simulink model "Quaternions_Method"  (R2021b)
settings: Solver=ode113  StartTime=0.0  StopTime=Time  RelTol=1e-13  AbsTol=1e-8
undefined symbols (not defined in the file): a, A_MB, A_SP, c, e, I, ii, Iinv, Ix, Iy, Iz, muP, om_x, om_y, om_z, omega_0, RS_MB, Rs_SP, theta00
libraries: vrlib x3, matrix_library x3, simulink_extras x1, robotcorelib x1
settings Model: Creator=dario  LastModifiedBy=adity
settings SolverCC: InitialStep=1e-3  AlgebraicLoopSolver=TrustRegion

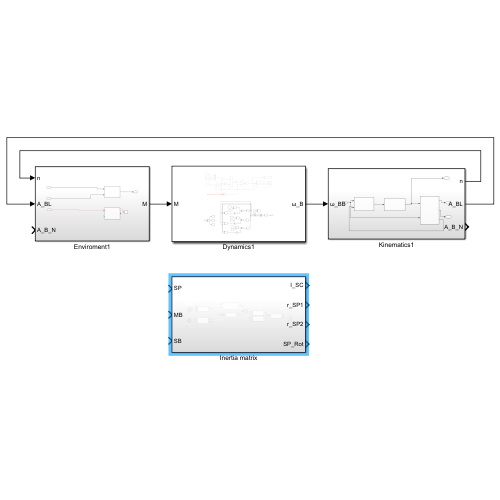
[thumbnail: Simulink's stored preview of the top-level diagram]
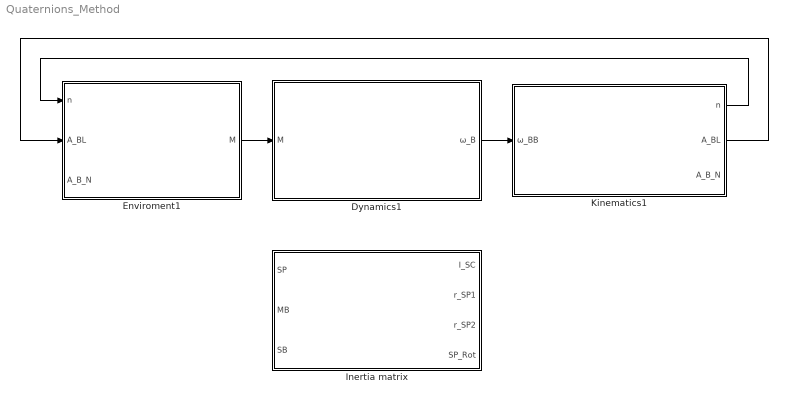
== system Quaternions_Method ==
  Dynamics1 : Subsystem
  Enviroment1 : Subsystem
  Inertia matrix : Subsystem
  Kinematics1 : Subsystem
  wires:
  Kinematics1/1(n) -> Enviroment1/1(n)
  Kinematics1/2(A_BL) -> Enviroment1/2(A_BL)
  Dynamics1/1(ω_B) -> Kinematics1/1(ω_BB)
  Enviroment1/1(M) -> Dynamics1/1(M)

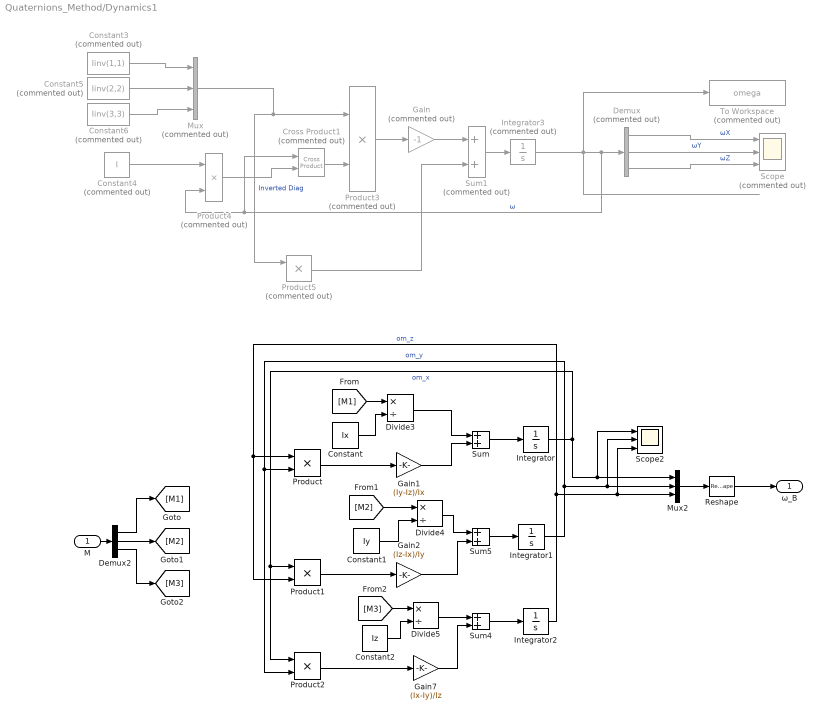
== system Quaternions_Method/Dynamics1 ==
  M : Inport
  Constant : Constant  Value=Ix
  Constant1 : Constant  Value=Iy
  Constant2 : Constant  Value=Iz
  Constant3 : Constant  Commented=on  Value=Iinv(1,1)
  Constant4 : Constant  Commented=on  Value=I
  Constant5 : Constant  Commented=on  Value=Iinv(2,2)
  Constant6 : Constant  Commented=on  Value=Iinv(3,3)
  Cross Product1 : vrlib/Utilities/Cross Product  Commented=on
  Demux : Demux  Commented=on  Outputs=3
  Demux2 : Demux  Outputs=3
  Divide3 : Product  Inputs=*/
  Divide4 : Product  Inputs=*/
  Divide5 : Product  Inputs=*/
  Gain : Gain  Commented=on  Gain=-1
  Gain1 : Gain  Gain=(Iy-Iz)/Ix
  Gain2 : Gain  Gain=(Iz-Ix)/Iy
  Gain7 : Gain  Gain=(Ix-Iy)/Iz
  Integrator : Integrator  InitialCondition=om_x
  Integrator1 : Integrator  InitialCondition=om_y
  Integrator2 : Integrator  InitialCondition=om_z
  Integrator3 : Integrator  Commented=on  InitialCondition=omega_0
  Mux : Mux  Commented=on  Inputs=3
  Mux2 : Mux  Inputs=3
  Product : Product
  Product1 : Product
  Product2 : Product
  Product3 : Product  Commented=on
  Product4 : Product  Commented=on
  Product5 : Product  Commented=on
  Reshape : Reshape  OutputDimensionality=Column vector (2-D)
  Scope : Scope  Commented=on  NumInputPorts=3
  Scope2 : Scope  NumInputPorts=3
  Sum : Sum  Inputs=|+|+|
  Sum1 : Sum  Commented=on
  Sum4 : Sum  Inputs=|+|+|
  Sum5 : Sum  Inputs=|+|+|
  To Workspace : ToWorkspace  Commented=on  VariableName=omega  SaveFormat=Timeseries  SampleTime=-1
  ω_B : Outport
  wires:
  Demux2/2 -> [M2]
  Demux2/3 -> [M3]
  Demux2/1 -> [M1]
  M/1 -> Demux2/1
  Integrator/1 -> Product2/1, Product1/1, Scope2/1, Mux2/1  "om_x"
  Integrator1/1 -> Scope2/2, Mux2/2, Product2/2, Product/2  "om_y"
  Integrator2/1 -> Mux2/3, Scope2/3, Product1/2, Product/1  "om_z"
  [M1] -> Divide3/1
  Constant/1 -> Divide3/2
  Product/1 -> Gain1/1
  Gain1/1 -> Sum/2
  Divide3/1 -> Sum/1
  Sum/1 -> Integrator/1
  [M2] -> Divide4/1
  Constant1/1 -> Divide4/2
  Divide4/1 -> Sum5/1
  Product1/1 -> Gain2/1
  Gain2/1 -> Sum5/2
  Sum5/1 -> Integrator1/1
  [M3] -> Divide5/1
  Constant2/1 -> Divide5/2
  Divide5/1 -> Sum4/1
  Sum4/1 -> Integrator2/1
  Product2/1 -> Gain7/1
  Gain7/1 -> Sum4/2
  Integrator3/1 -> To Workspace/1, Demux/1, Product4/2, Cross Product1/1  "ω"
  Sum1/1 -> Integrator3/1
  Mux/1 -> Product5/1, Product3/1  "Inverted Diag"
  Constant6/1 -> Mux/3
  Gain/1 -> Sum1/1
  Cross Product1/1 -> Product3/2
  Product3/1 -> Gain/1
  ? -> Product5/2
  Product5/1 -> Sum1/2
  Demux/2 -> Scope/2  "ωY"
  Constant3/1 -> Mux/1
  Constant5/1 -> Mux/2
  Product4/1 -> Cross Product1/2
  Constant4/1 -> Product4/1
  Demux/1 -> Scope/1  "ωX"
  Demux/3 -> Scope/3  "ωZ"
  Mux2/1 -> Reshape/1
  Reshape/1 -> ω_B/1

== system Quaternions_Method/Enviroment1 ==
  n : Inport
  A_BL : Inport  Port=2
  A_B_N : Inport  Port=3
  Gravity_Gradient : Subsystem
  Solar Radiation Perturbation : Subsystem
  Terminator : Terminator
  M : Outport
  wires:
  A_BL/1 -> Gravity_Gradient/1(A_BL)
  Gravity_Gradient/1(M_GG) -> M/1
  n/1 -> Gravity_Gradient/2(n)
  ? -> Terminator/1
  A_B_N/1 -> ?

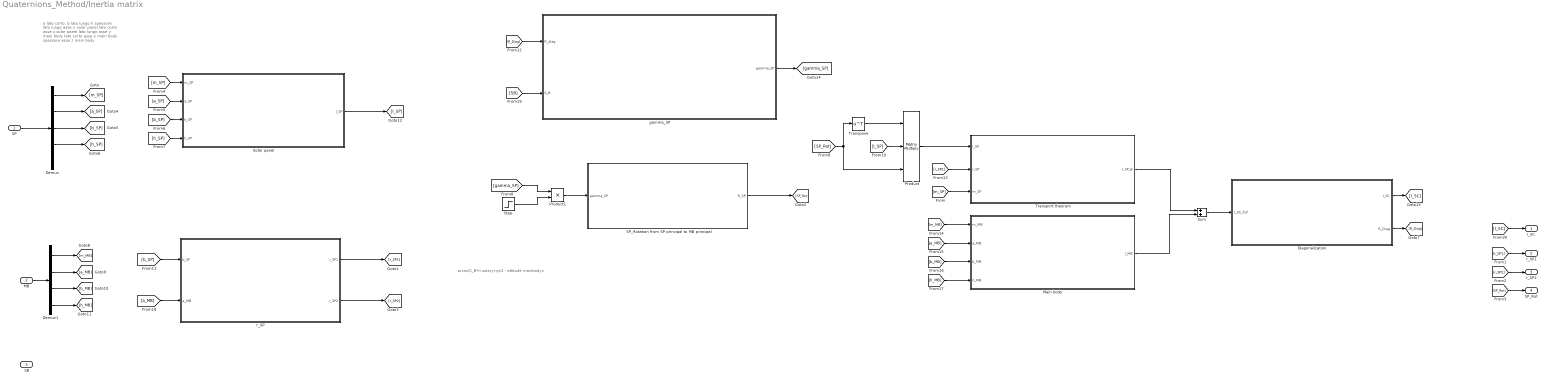
== system Quaternions_Method/Inertia matrix ==
  note: arcos(S_B*n solary)-pi/2 - attitude mainbodyx
  note: a lato corto, b lato lungo h spessore
      | lato lungo asse x solar panel
      | lato corto asse z solar panel
      | lato lungo asse y main body
      | lato corto asse x main body
      | spessore asse z main body
  SP : Inport
  MB : Inport  Port=2
  SB : Inport  Port=3
  Demux : Demux  Outputs=5
  Demux1 : Demux
  Diagonalization : Subsystem
  Main body : Subsystem
  Product : Product  Inputs=3  Multiplication=Matrix(*)
  Product1 : Product
  SP_Rotation from SP principal to MB principal : Subsystem
  Solar panel : Subsystem
  Step : Step  Time=1e-3  SampleTime=0
  Sum : Sum
  Transport theorem : Subsystem
  Transpose : Math  Operator=transpose  SaturateOnIntegerOverflow=on
  gamma_SP : Subsystem
  r_SP : Subsystem
  I_SC : Outport
  r_SP1 : Outport  Port=2
  r_SP2 : Outport  Port=3
  SP_Rot : Outport  Port=4
  wires:
  MB/1 -> Demux1/1
  Demux/1 -> [m_SP]
  Product/1 -> Transport theorem/1(I_SP)
  SP_Rotation from SP principal to MB principal/1(R_SP) -> [SP_Rot]
  Transpose/1 -> Product/1
  Transport theorem/1(I_SP_B) -> Sum/1
  [r_SP1] -> Transport theorem/2(r_SP)
  Sum/1 -> Diagonalization/1(I_SC_full)
  Main body/1(I_MB) -> Sum/2
  [m_SP] -> Transport theorem/3(m_SP)
  r_SP/1(r_SP1) -> [r_SP1]
  [r_SP1] -> r_SP1/1
  [r_SP2] -> r_SP2/1
  [SP_Rot] -> SP_Rot/1
  r_SP/2(r_SP2) -> [r_SP2]
  Demux/2 -> [a_SP]
  Demux/3 -> [b_SP]
  Demux/4 -> [h_SP]
  [a_SP] -> Solar panel/2(a_SP)
  [b_SP] -> Solar panel/3(b_SP)
  [m_SP] -> Solar panel/1(m_SP)
  [h_SP] -> Solar panel/4(h_SP)
  [SP_Rot] -> Transpose/1, Product/3
  [b_SP] -> r_SP/1(b_SP)
  Demux1/4 -> [h_MB]
  Demux1/3 -> [b_MB]
  Demux1/2 -> [a_MB]
  Demux1/1 -> [m_MB]
  [m_MB] -> Main body/1(m_MB)
  [a_MB] -> Main body/2(a_MB)
  [b_MB] -> Main body/3(b_MB)
  [h_MB] -> Main body/4(h_MB)
  [a_MB] -> r_SP/2(a_MB)
  Solar panel/1(I_SP) -> [I_SP]
  [I_SP] -> Product/2
  Product1/1 -> SP_Rotation from SP principal to MB principal/1(gamma_SP)
  [gamma_SP] -> Product1/1
  Step/1 -> Product1/2
  SP/1 -> Demux/1
  Diagonalization/2(R_Diag) -> [R_Diag]
  [R_Diag] -> gamma_SP/1(R_diag)
  [SB] -> gamma_SP/2(S_B)
  Diagonalization/1(I_SC) -> [I_SC]
  [I_SC] -> I_SC/1
  gamma_SP/1(gamma_SP) -> [gamma_SP]

== system Quaternions_Method/Kinematics1 ==
  ω_BB : Inport
  Creazione Matrice A_BN : Subsystem
  Creazione quaternione : Subsystem
  Relative_Attitude : Subsystem
  n : Outport
  A_BL : Outport  Port=2
  A_B_N : Outport  Port=3
  wires:
  Creazione Matrice A_BN/1(A_BN) -> A_B_N/1, Relative_Attitude/1(A_BN)
  ω_BB/1 -> Relative_Attitude/2(ω_BB), Creazione quaternione/1(ω_BB)
  Creazione quaternione/1(q_normalizzato) -> Creazione Matrice A_BN/1(q_normalizzato)
  Relative_Attitude/1(A_BL) -> A_BL/1
  Relative_Attitude/2(n) -> n/1
  Relative_Attitude/3(A_L/N) -> Creazione quaternione/2(A_LN)

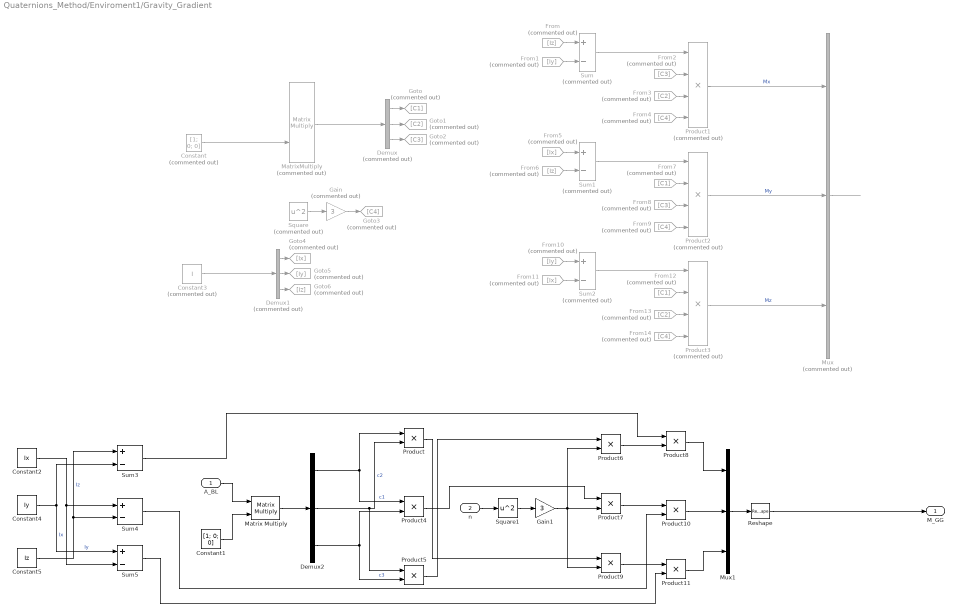
== system Quaternions_Method/Enviroment1/Gravity_Gradient ==
  A_BL : Inport
  n : Inport  Port=2
  Constant : Constant  Commented=on  Value=[1; 0; 0]
  Constant1 : Constant  Value=[1; 0; 0]
  Constant2 : Constant  Value=Ix
  Constant3 : Constant  Commented=on  Value=I
  Constant4 : Constant  Value=Iy
  Constant5 : Constant  Value=Iz
  Demux : Demux  Commented=on  Outputs=3
  Demux1 : Demux  Commented=on  Outputs=3
  Demux2 : Demux  Outputs=3
  From : From  Commented=on  GotoTag=Iz
  From1 : From  Commented=on  GotoTag=Iy
  From10 : From  Commented=on  GotoTag=Iy
  From11 : From  Commented=on  GotoTag=Ix
  From12 : From  Commented=on  GotoTag=C1
  From13 : From  Commented=on  GotoTag=C2
  From14 : From  Commented=on  GotoTag=C4
  From2 : From  Commented=on  GotoTag=C3
  From3 : From  Commented=on  GotoTag=C2
  From4 : From  Commented=on  GotoTag=C4
  From5 : From  Commented=on  GotoTag=Ix
  From6 : From  Commented=on  GotoTag=Iz
  From7 : From  Commented=on  GotoTag=C1
  From8 : From  Commented=on  GotoTag=C3
  From9 : From  Commented=on  GotoTag=C4
  Gain : Gain  Commented=on  Gain=3
  Gain1 : Gain  Gain=3
  Goto : Goto  Commented=on  GotoTag=C1
  Goto1 : Goto  Commented=on  GotoTag=C2
  Goto2 : Goto  Commented=on  GotoTag=C3
  Goto3 : Goto  Commented=on  GotoTag=C4
  Goto4 : Goto  Commented=on  GotoTag=Ix
  Goto5 : Goto  Commented=on  GotoTag=Iy
  Goto6 : Goto  Commented=on  GotoTag=Iz
  Matrix Multiply : Product  Multiplication=Matrix(*)
  MatrixMultiply : Product  Commented=on  Multiplication=Matrix(*)
  Mux : Mux  Commented=on  Inputs=3
  Mux1 : Mux  Inputs=3
  Product{,4..11} (9 alike) : Product
  Product1 : Product  Commented=on  Inputs=4
  Product2 : Product  Commented=on  Inputs=4
  Product3 : Product  Commented=on  Inputs=4
  Reshape : Reshape  OutputDimensionality=Column vector (2-D)
  Square : Math  Commented=on  Operator=square  SaturateOnIntegerOverflow=on
  Square1 : Math  Operator=square  SaturateOnIntegerOverflow=on
  Sum : Sum  Commented=on  Inputs=+-
  Sum1 : Sum  Commented=on  Inputs=+-
  Sum2 : Sum  Commented=on  Inputs=+-
  Sum3 : Sum  Inputs=|+|-|
  Sum4 : Sum  Inputs=|+|-|
  Sum5 : Sum  Inputs=|+|-|
  M_GG : Outport
  wires:
  Constant/1 -> MatrixMultiply/2
  MatrixMultiply/1 -> Demux/1
  Constant3/1 -> Demux1/1
  Product1/1 -> Mux/1  "Mx"
  Product2/1 -> Mux/2  "My"
  Demux/1 -> Goto/1
  Demux/2 -> Goto1/1
  Demux/3 -> Goto2/1
  Demux1/1 -> Goto4/1
  Demux1/2 -> Goto5/1
  Demux1/3 -> Goto6/1
  From/1 -> Sum/1
  From1/1 -> Sum/2
  Sum/1 -> Product1/1
  From2/1 -> Product1/2
  From3/1 -> Product1/3
  From4/1 -> Product1/4
  From5/1 -> Sum1/1
  From6/1 -> Sum1/2
  Sum1/1 -> Product2/1
  From7/1 -> Product2/2
  From8/1 -> Product2/3
  From9/1 -> Product2/4
  From10/1 -> Sum2/1
  From14/1 -> Product3/4
  From12/1 -> Product3/2
  From13/1 -> Product3/3
  Sum2/1 -> Product3/1
  From11/1 -> Sum2/2
  Product3/1 -> Mux/3  "Mz"
  Square/1 -> Gain/1
  Gain/1 -> Goto3/1
  A_BL/1 -> Matrix Multiply/1
  Constant1/1 -> Matrix Multiply/2
  Matrix Multiply/1 -> Demux2/1
  Demux2/1 -> Product4/1, Product/1  "c1"
  Demux2/3 -> Product5/2, Product4/2  "c3"
  Demux2/2 -> Product5/1, Product/2  "c2"
  Constant5/1 -> Sum4/2, Sum3/1  "Iz"
  Constant4/1 -> Sum3/2, Sum5/1  "Iy"
  Constant2/1 -> Sum5/2, Sum4/1  "Ix"
  n/1 -> Square1/1
  Square1/1 -> Gain1/1
  Product5/1 -> Product6/1
  Gain1/1 -> Product9/2, Product7/2, Product6/2
  Product4/1 -> Product7/1
  Product/1 -> Product9/1
  Sum3/1 -> Product8/1
  Product6/1 -> Product8/2
  Product7/1 -> Product10/1
  Sum4/1 -> Product10/2
  Sum5/1 -> Product11/2
  Product9/1 -> Product11/1
  Product10/1 -> Mux1/2
  Product8/1 -> Mux1/1
  Product11/1 -> Mux1/3
  ? -> MatrixMultiply/1
  ? -> Square/1
  Mux/1 -> ?
  Mux1/1 -> Reshape/1
  Reshape/1 -> M_GG/1

== system Quaternions_Method/Enviroment1/Solar Radiation Perturbation ==
  n_SP : Inport
  A_B_N : Inport  Port=2
  Constant : Constant  Value=A_SP
  Constant1 : Constant  Value=Rs_SP
  Constant2 : Constant  Value=RS_MB
  Constant3 : Constant  Value=A_MB
  Constant6 : Constant  Value=1358
  Constant7 : Constant  Value=c
  Force : Subsystem
  From Workspace1 : FromWorkspace  VariableName=Rd
  N_MB : Constant  Value=[1 0 0;0 1 0;0 0 1]
  Normalize Vector : vrlib/Utilities/Normalize Vector  maxzero=0
  Product : Product
  Reciprocal : Product  Inputs=1
  Sum forces : Subsystem
  Sun position body : Subsystem
  Output : Outport
  wires:
  From Workspace1/1 -> Force/9(R_D)
  Constant/1 -> Force/7(A_SP)
  n_SP/1 -> Force/6(n_SP)
  Constant7/1 -> Reciprocal/1
  Constant6/1 -> Product/1
  Constant3/1 -> Force/3(A_MB)
  Constant2/1 -> Force/2(RS_MB)
  N_MB/1 -> Force/5(N_MB)
  Constant1/1 -> Force/8(Rs_SP)
  Normalize Vector/1 -> Force/4(SB)
  Reciprocal/1 -> Product/2
  Product/1 -> Force/1(P)
  A_B_N/1 -> Sun position body/1(A_B_N)
  Sun position body/1(S_B) -> Normalize Vector/1

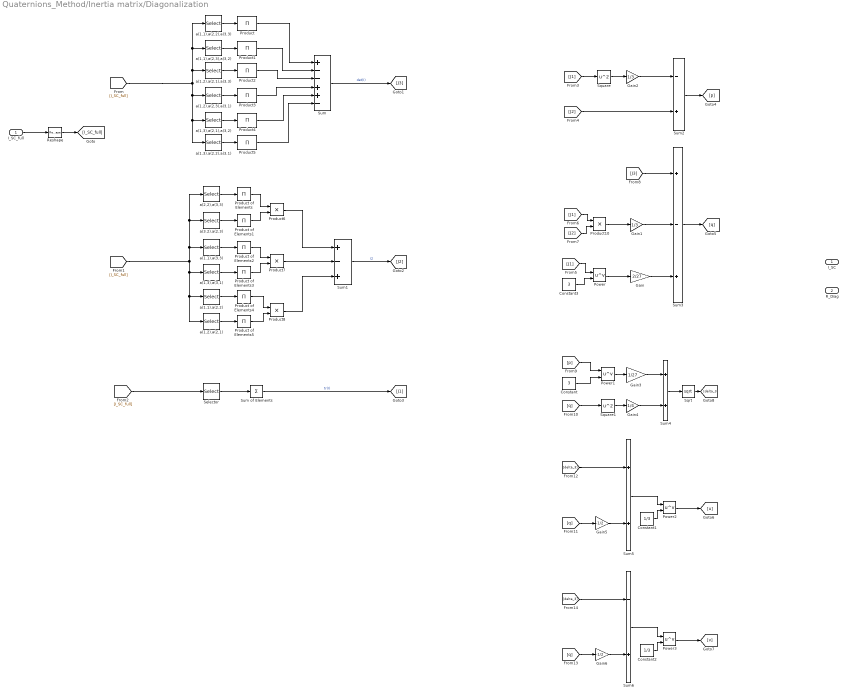
== system Quaternions_Method/Inertia matrix/Diagonalization ==
  I_SC_full : Inport
  Constant : Constant  Value=3
  Constant1 : Constant  Value=1/3
  Constant2 : Constant  Value=1/3
  Constant3 : Constant  Value=3
  Gain : Gain  Gain=2/27
  Gain1 : Gain  Gain=1/3
  Gain2 : Gain  Gain=1/3
  Gain3 : Gain  Gain=1/27
  Gain4 : Gain  Gain=1/4
  Gain5 : Gain  Gain=-1/2
  Gain6 : Gain  Gain=-1/2
  Power{,1..3} (4 alike) : Math  Operator=pow  SaturateOnIntegerOverflow=on
  Product{,1..5} (6 alike) : Product  Inputs=1  SaturateOnIntegerOverflow=on  OutDataTypeStr=Inherit: Same as first input
  Product of Elements{,1..5} (6 alike) : Product  Inputs=*
  Product{6..8,10} (4 alike) : Product
  Reshape : Reshape  OutputDimensionality=Column vector (2-D)
  Selector : Selector  InputPortWidth=9  IndexOptions=Index vector (dialog)  Indices=[1 5 9]  OutputSizes=1
  Sqrt : Sqrt  SaturateOnIntegerOverflow=on
  Square : Math  Operator=square  SaturateOnIntegerOverflow=on
  Square1 : Math  Operator=square  SaturateOnIntegerOverflow=on
  Sum : Sum  Inputs=+--++-  SaturateOnIntegerOverflow=on
  Sum of Elements : Sum  Inputs=+
  Sum1 : Sum  Inputs=+-+
  Sum2 : Sum  Inputs=-+
  Sum3 : Sum  Inputs=+-+
  Sum4 : Sum
  Sum5 : Sum
  Sum6 : Sum  Inputs=-+
  a(1,1),a(2,2) : Selector  InputPortWidth=9  IndexOptions=Index vector (dialog)  Indices=[1 3]  OutputSizes=1
  a(1,1),a(2,2),a(3,3) : Selector  InputPortWidth=9  IndexOptions=Index vector (dialog)  Indices=[1 5 9]  OutputSizes=1
  a(1,1),a(2,3),a(3,2) : Selector  InputPortWidth=9  IndexOptions=Index vector (dialog)  Indices=[1 6 8]  OutputSizes=1
  a(1,2),a(2,1) : Selector  InputPortWidth=9  IndexOptions=Index vector (dialog)  Indices=[1 3]  OutputSizes=1
  a(1,2),a(2,1),a(3,3) : Selector  InputPortWidth=9  IndexOptions=Index vector (dialog)  Indices=[2 4 9]  OutputSizes=1
  a(1,2),a(2,3),a(3,1) : Selector  InputPortWidth=9  IndexOptions=Index vector (dialog)  Indices=[3 4 8]  OutputSizes=1
  a(1,3),a(2,1),a(3,2) : Selector  InputPortWidth=9  IndexOptions=Index vector (dialog)  Indices=[2 6 7]  OutputSizes=1
  a(1,3),a(2,2),a(3,1) : Selector  InputPortWidth=9  IndexOptions=Index vector (dialog)  Indices=[3 5 7]  OutputSizes=1
  a(1,3),a(3,1) : Selector  InputPortWidth=9  IndexOptions=Index vector (dialog)  Indices=[1 3]  OutputSizes=1
  a(1.1),a(3,3) : Selector  InputPortWidth=9  IndexOptions=Index vector (dialog)  Indices=[1 3]  OutputSizes=1
  a(2,2),a(3,3) : Selector  InputPortWidth=9  IndexOptions=Index vector (dialog)  Indices=[5 9]  OutputSizes=1
  a(3.2),a(2,3) : Selector  InputPortWidth=9  IndexOptions=Index vector (dialog)  Indices=[6 8]  OutputSizes=1
  I_SC : Outport
  R_Diag : Outport  Port=2
  wires:
  [I_SC_full] -> a(1,3),a(2,2),a(3,1)/1, a(1,3),a(2,1),a(3,2)/1, a(1,2),a(2,3),a(3,1)/1, a(1,1),a(2,2),a(3,3)/1, a(1,1),a(2,3),a(3,2)/1, a(1,2),a(2,1),a(3,3)/1
  Product2/1 -> Sum/3
  Product3/1 -> Sum/4
  a(1,2),a(2,1),a(3,3)/1 -> Product2/1
  a(1,1),a(2,3),a(3,2)/1 -> Product1/1
  Product/1 -> Sum/1
  a(1,3),a(2,2),a(3,1)/1 -> Product5/1
  a(1,1),a(2,2),a(3,3)/1 -> Product/1
  a(1,3),a(2,1),a(3,2)/1 -> Product4/1
  Product4/1 -> Sum/5
  Product1/1 -> Sum/2
  Product5/1 -> Sum/6
  a(1,2),a(2,3),a(3,1)/1 -> Product3/1
  I_SC_full/1 -> Reshape/1
  Reshape/1 -> [I_SC_full]
  Sum/1 -> [J3]  "det(I)"
  Product6/1 -> Sum1/1
  Product7/1 -> Sum1/2
  Product8/1 -> Sum1/3
  Sum1/1 -> [J2]  "I2"
  [I_SC_full] -> a(1,3),a(3,1)/1, a(1,1),a(2,2)/1, a(1,2),a(2,1)/1, a(1.1),a(3,3)/1, a(3.2),a(2,3)/1, a(2,2),a(3,3)/1
  [I_SC_full] -> Selector/1
  Selector/1 -> Sum of Elements/1
  a(2,2),a(3,3)/1 -> Product of Elements/1
  a(3.2),a(2,3)/1 -> Product of Elements1/1
  a(1.1),a(3,3)/1 -> Product of Elements2/1
  a(1,3),a(3,1)/1 -> Product of Elements3/1
  a(1,1),a(2,2)/1 -> Product of Elements4/1
  a(1,2),a(2,1)/1 -> Product of Elements5/1
  Product of Elements5/1 -> Product8/2
  Product of Elements4/1 -> Product8/1
  Product of Elements3/1 -> Product7/2
  Product of Elements2/1 -> Product7/1
  Product of Elements1/1 -> Product6/2
  Product of Elements/1 -> Product6/1
  Sum of Elements/1 -> [J1]  "tr(I)"
  [J2] -> Sum2/2
  [J1] -> Square/1
  Square/1 -> Gain2/1
  Gain2/1 -> Sum2/1
  Sum2/1 -> [p]
  [J2] -> Product10/2
  [J1] -> Product10/1
  [J3] -> Sum3/1
  Constant3/1 -> Power/2
  [J1] -> Power/1
  Power/1 -> Gain/1
  Product10/1 -> Gain1/1
  Gain1/1 -> Sum3/2
  Gain/1 -> Sum3/3
  Sum3/1 -> [q]
  [q] -> Square1/1
  [p] -> Power1/1
  Constant/1 -> Power1/2
  Square1/1 -> Gain4/1
  Power1/1 -> Gain3/1
  Gain4/1 -> Sum4/2
  Gain3/1 -> Sum4/1
  Sum4/1 -> Sqrt/1
  [q] -> Gain5/1
  Gain5/1 -> Sum5/2
  Sum5/1 -> Power2/1
  Constant1/1 -> Power2/2
  Power2/1 -> [u]
  Sqrt/1 -> [delta_3]
  [delta_3] -> Sum5/1
  [delta_3] -> Sum6/1
  Constant2/1 -> Power3/2
  Sum6/1 -> Power3/1
  [q] -> Gain6/1
  Power3/1 -> [v]
  Gain6/1 -> Sum6/2

== system Quaternions_Method/Inertia matrix/Main body ==
  m_MB : Inport
  a_MB : Inport  Port=2
  b_MB : Inport  Port=3
  h_MB : Inport  Port=4
  Gain : Gain  Gain=1/12
  Gain1 : Gain  Gain=1/12
  Gain2 : Gain  Gain=1/12
  Ground : Ground
  Product : Product
  Product1 : Product
  Product2 : Product
  Reshape : Reshape  OutputDimensionality=Customize  OutputDimensions=[3,3]
  Square : Math  Operator=square  SaturateOnIntegerOverflow=on
  Square1 : Math  Operator=square  SaturateOnIntegerOverflow=on
  Square2 : Math  Operator=square  SaturateOnIntegerOverflow=on
  Sum : Sum
  Sum1 : Sum
  Sum2 : Sum
  Vector Concatenate : Concatenate  NumInputs=9
  I_MB : Outport
  wires:
  Ground/1 -> Vector Concatenate/2, Vector Concatenate/3, Vector Concatenate/7, Vector Concatenate/8, Vector Concatenate/6, Vector Concatenate/4
  Square/1 -> Sum2/1, Sum1/1
  Square1/1 -> Sum2/2, Sum/1
  Square2/1 -> Sum/2, Sum1/2
  Product1/1 -> Gain1/1
  Gain/1 -> Vector Concatenate/1
  Product2/1 -> Gain2/1
  Sum1/1 -> Product1/2
  m_MB/1 -> Product/1, Product2/1, Product1/1
  Sum2/1 -> Product2/2
  a_MB/1 -> Square/1
  Vector Concatenate/1 -> Reshape/1
  Sum/1 -> Product/2
  b_MB/1 -> Square1/1
  Gain1/1 -> Vector Concatenate/5
  Product/1 -> Gain/1
  Gain2/1 -> Vector Concatenate/9
  Reshape/1 -> I_MB/1
  h_MB/1 -> Square2/1

== system Quaternions_Method/Inertia matrix/SP_Rotation from SP principal to MB principal ==
  gamma_SP : Inport
  Constant : Constant
  Gain : Gain  Gain=-1
  Ground : Ground
  Reshape : Reshape  OutputDimensionality=Customize  OutputDimensions=[3,3]
  Sin : Trigonometry  Operator=cos
  Sin1 : Trigonometry
  Vector Concatenate : Concatenate  NumInputs=9
  R_SP : Outport
  wires:
  Vector Concatenate/1 -> Reshape/1
  Reshape/1 -> R_SP/1
  Constant/1 -> Vector Concatenate/1
  Ground/1 -> Vector Concatenate/7, Vector Concatenate/4, Vector Concatenate/3, Vector Concatenate/2
  gamma_SP/1 -> Sin1/1, Sin/1
  Gain/1 -> Vector Concatenate/6
  Sin/1 -> Vector Concatenate/5, Vector Concatenate/9
  Sin1/1 -> Gain/1, Vector Concatenate/8

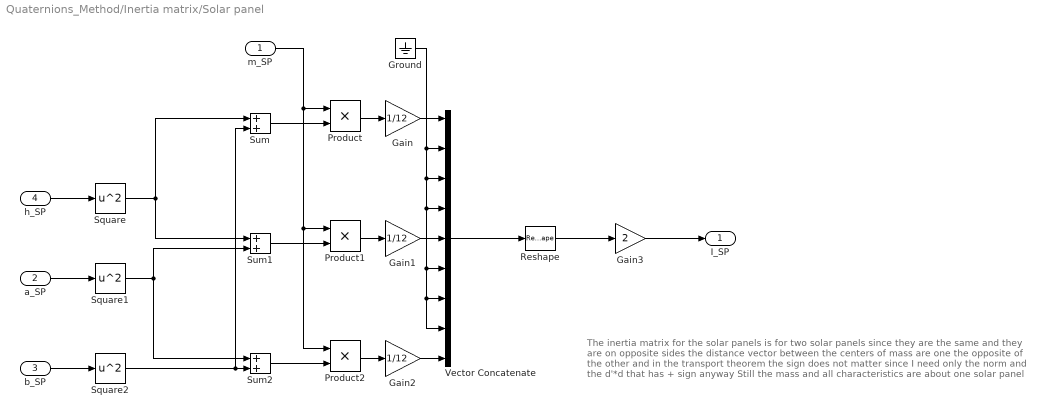
== system Quaternions_Method/Inertia matrix/Solar panel ==
  note: The inertia matrix for the solar panels is for two solar panels since they are the same and they are on opposite sides the distance vector between the centers of mass are one the opposite of the other and in the transport theorem the sign does not matter since I need only the norm and the d'*d that has + sign anyway
      | Still the mass and all characteristics are about one solar panel
  m_SP : Inport
  a_SP : Inport  Port=2
  b_SP : Inport  Port=3
  h_SP : Inport  Port=4
  Gain : Gain  Gain=1/12
  Gain1 : Gain  Gain=1/12
  Gain2 : Gain  Gain=1/12
  Gain3 : Gain  Gain=2
  Ground : Ground
  Product : Product
  Product1 : Product
  Product2 : Product
  Reshape : Reshape  OutputDimensionality=Customize  OutputDimensions=[3,3]
  Square : Math  Operator=square  SaturateOnIntegerOverflow=on
  Square1 : Math  Operator=square  SaturateOnIntegerOverflow=on
  Square2 : Math  Operator=square  SaturateOnIntegerOverflow=on
  Sum : Sum
  Sum1 : Sum
  Sum2 : Sum
  Vector Concatenate : Concatenate  NumInputs=9
  I_SP : Outport
  wires:
  Vector Concatenate/1 -> Reshape/1
  m_SP/1 -> Product/1, Product2/1, Product1/1
  Product/1 -> Gain/1
  Gain/1 -> Vector Concatenate/1
  Product1/1 -> Gain1/1
  Product2/1 -> Gain2/1
  Gain2/1 -> Vector Concatenate/9
  h_SP/1 -> Square/1
  a_SP/1 -> Square1/1
  b_SP/1 -> Square2/1
  Sum/1 -> Product/2
  Sum1/1 -> Product1/2
  Sum2/1 -> Product2/2
  Ground/1 -> Vector Concatenate/2, Vector Concatenate/3, Vector Concatenate/7, Vector Concatenate/8, Vector Concatenate/6, Vector Concatenate/4
  Gain1/1 -> Vector Concatenate/5
  Reshape/1 -> Gain3/1
  Gain3/1 -> I_SP/1
  Square1/1 -> Sum1/2, Sum2/1
  Square2/1 -> Sum/2, Sum2/2
  Square/1 -> Sum/1, Sum1/1

== system Quaternions_Method/Inertia matrix/Transport theorem ==
  I_SP : Inport
  r_SP : Inport  Port=2
  m_SP : Inport  Port=3
  Constant : Constant  Value=eye(3)
  Dot Product : DotProduct  InputSameDT=on  OutDataTypeStr=Inherit: Inherit via internal rule
  Gain : Gain  Gain=2
  Matrix Multiply : Product  Multiplication=Matrix(*)
  Matrix Multiply1 : Product
  Product : Product
  Sum : Sum  Inputs=+-
  Sum1 : Sum
  Transpose : Math  Operator=transpose  SaturateOnIntegerOverflow=on
  I_SP_B : Outport
  wires:
  r_SP/1 -> Transpose/1, Dot Product/2, Dot Product/1, Matrix Multiply/2
  Transpose/1 -> Matrix Multiply/1
  Constant/1 -> Matrix Multiply1/1
  Matrix Multiply1/1 -> Sum/1
  Matrix Multiply/1 -> Sum/2
  Sum/1 -> Product/2
  m_SP/1 -> Gain/1
  Product/1 -> Sum1/2
  I_SP/1 -> Sum1/1
  Sum1/1 -> I_SP_B/1
  Dot Product/1 -> Matrix Multiply1/2
  Gain/1 -> Product/1

== system Quaternions_Method/Inertia matrix/gamma_SP ==
  R_diag : Inport
  S_B : Inport  Port=2
  Cos : Trigonometry  Operator=acos
  Demux : Demux  Outputs=3
  Gain : Gain  Gain=-1
  Matrix Multiply1 : Product  Multiplication=Matrix(*)
  Terminator : Terminator
  Terminator1 : Terminator
  gamma_SP : Outport
  wires:
  R_diag/1 -> Matrix Multiply1/1
  S_B/1 -> Matrix Multiply1/2
  Matrix Multiply1/1 -> Demux/1  "S_p_SP"
  Demux/1 -> Terminator/1
  Demux/2 -> Terminator1/1
  Demux/3 -> Gain/1
  Gain/1 -> Cos/1
  Cos/1 -> gamma_SP/1

== system Quaternions_Method/Inertia matrix/r_SP ==
  b_SP : Inport
  a_MB : Inport  Port=2
  Constant : Constant  Value=[1 0 0]
  Gain : Gain  Gain=1/2
  Gain1 : Gain  Gain=1/2
  Gain2 : Gain  Gain=-1
  Product : Product
  Reshape : Reshape  OutputDimensionality=Column vector (2-D)
  Sum : Sum
  r_SP1 : Outport
  r_SP2 : Outport  Port=2
  wires:
  Constant/1 -> Reshape/1
  a_MB/1 -> Gain/1
  b_SP/1 -> Gain1/1
  Gain1/1 -> Sum/1
  Gain/1 -> Sum/2
  Reshape/1 -> Product/1
  Sum/1 -> Product/2
  Gain2/1 -> r_SP2/1
  Product/1 -> r_SP1/1, Gain2/1

== system Quaternions_Method/Kinematics1/Creazione Matrice A_BN ==
  q_normalizzato : Inport
  Matrix Concatenate : Concatenate  NumInputs=3  Mode=Multidimensional array  ConcatenateDimension=2
  Scope : Scope
  column 1 : Subsystem
  column 2 : Subsystem
  column 3 : Subsystem
  A_BN : Outport
  wires:
  Matrix Concatenate/1 -> Scope/1, A_BN/1
  q_normalizzato/1 -> column 3/1(q_normalizzato), column 1/1(q_normalizzato), column 2/1(q_normalizzato)
  column 1/1(Column 1) -> Matrix Concatenate/1
  column 2/1(Column 2) -> Matrix Concatenate/2
  column 3/1(Column 3) -> Matrix Concatenate/3

== system Quaternions_Method/Kinematics1/Creazione quaternione ==
  ω_BB : Inport
  A_LN : Inport  Port=2
  Creation matrix [OM] : MATLAB Function  TreatAsAtomicUnit=on
  Demux : Demux  Outputs=3
  Gain : Gain  Gain=0.5
  Initial condition quaternion : Subsystem
  Integrator : Integrator  InitialConditionSource=external  InitialCondition=[0; 0; 0; 1]
  Matrix Multiply : Product  Multiplication=Matrix(*)
  Normalisation : Subsystem
  Reshape : Reshape  OutputDimensionality=Column vector (2-D)
  q_normalizzato : Outport
  wires:
  Creation matrix [OM]/1(OM) -> Gain/1
  Matrix Multiply/1 -> Integrator/1  "dq/dt"
  Gain/1 -> Matrix Multiply/1
  ω_BB/1 -> Demux/1
  Demux/1 -> Creation matrix [OM]/1(om_x)
  Demux/2 -> Creation matrix [OM]/2(om_y)
  Demux/3 -> Creation matrix [OM]/3(om_z)
  Integrator/1 -> Reshape/1  "q(t)"
  Reshape/1 -> Normalisation/1(In1)
  A_LN/1 -> Initial condition quaternion/1(A_LN)
  Initial condition quaternion/1(Output) -> Integrator/2
  Normalisation/1(Out1) -> q_normalizzato/1, Matrix Multiply/2  "q(t)"

== system Quaternions_Method/Kinematics1/Relative_Attitude ==
  A_BN : Inport
  ω_BB : Inport  Port=2
  A_LN : Subsystem
  Constant : Constant  Value=0
  Coordinate Transformation Conversion : robotcorelib/Coordinate Transformation Conversion  InputRepresentation=Rotation Matrix  InputEulerSequence=ZYX  ShowTrVecInputPort=on  OutputRepresentation=Euler Angles  OutputEulerSequence=ZYX  ShowTrVecOutputPort=on  SimulateUsing=Interpreted execution
      settings: SourceProductBaseCode=NV,RO,RR,UV
  MatrixMultiply : Product  Multiplication=Matrix(*)
  MatrixMultiply1 : Product  Multiplication=Matrix(*)
  Mux : Mux  Inputs=3
  Orbit Propagation : Subsystem
  Reshape : Reshape  OutputDimensionality=Column vector (2-D)
  Scope : Scope
  Scope1 : Scope
  Sum : Sum  Inputs=-+
  Terminator : Terminator
  To Workspace : ToWorkspace  VariableName=A_BL  SaveFormat=Timeseries  SampleTime=-1
  To Workspace1 : ToWorkspace  VariableName=Omega_BL  SaveFormat=Timeseries  SampleTime=-1
  Transpose : Math  Operator=transpose  SaturateOnIntegerOverflow=on
  A_BL : Outport
  n : Outport  Port=2
  A_L/N : Outport  Port=3
  wires:
  Transpose/1 -> MatrixMultiply/2
  MatrixMultiply/1 -> To Workspace/1, Scope1/1, Coordinate Transformation Conversion/1, A_BL/1, MatrixMultiply1/1  "A_BL"
  A_LN/1(A_LN) -> A_L/N/1, Transpose/1
  A_BN/1 -> MatrixMultiply/1, Orbit Propagation/1(A_BN)
  ω_BB/1 -> Sum/2
  MatrixMultiply1/1 -> Sum/1
  Sum/1 -> Scope/1, To Workspace1/1  "ω_B/L"
  Orbit Propagation/1(n) -> Mux/3, n/1
  Mux/1 -> Reshape/1  "ω_LN"
  Constant/1 -> Mux/2, Mux/1
  Orbit Propagation/3(rB) -> Terminator/1
  Orbit Propagation/2(theta) -> A_LN/1(theta)
  Coordinate Transformation Conversion/1 -> ?
  Reshape/1 -> MatrixMultiply1/2

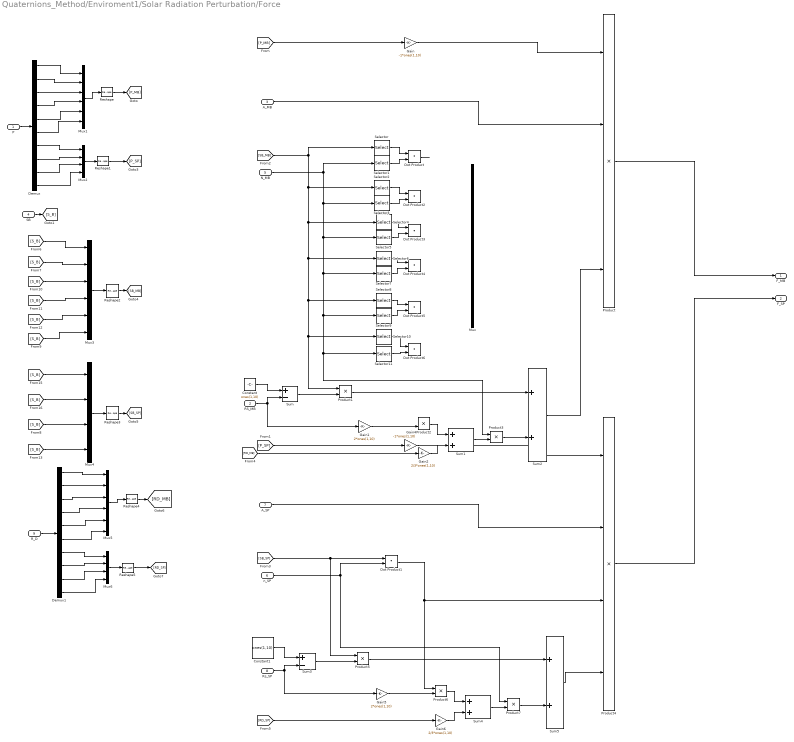
== system Quaternions_Method/Enviroment1/Solar Radiation Perturbation/Force ==
  P : Inport
  RS_MB : Inport  Port=2
  A_MB : Inport  Port=3
  SB : Inport  Port=4
  N_MB : Inport  Port=5
  n_SP : Inport  Port=6
  A_SP : Inport  Port=7
  Rs_SP : Inport  Port=8
  R_D : Inport  Port=9
  Constant : Constant  Value=ones(1,10)
  Constant1 : Constant  Value=ones(1,10)
  Demux : Demux  Outputs=10
  Demux1 : Demux  Outputs=10
  Dot Product{,1..6} (7 alike) : DotProduct  InputSameDT=on  OutDataTypeStr=Inherit: Inherit via internal rule
  Gain : Gain  Gain=-1*ones(1,10)
  Gain1 : Gain  Gain=2*ones(1,10)
  Gain2 : Gain  Gain=2/3*ones(1,10)
  Gain4 : Gain  Gain=-1*ones(1,10)
  Gain5 : Gain  Gain=2*ones(1,10)
  Gain6 : Gain  Gain=2/3*ones(1,10)
  Mux : Mux  Inputs=8
  Mux1 : Mux  Inputs=6
  Mux2 : Mux
  Mux3 : Mux  Inputs=6
  Mux4 : Mux
  Mux5 : Mux  Inputs=6
  Mux6 : Mux
  Product : Product  Inputs=4
  Product{1..3,5..7} (6 alike) : Product
  Product4 : Product  Inputs=4
  Reshape{,1,4..5} (4 alike) : Reshape  OutputDimensionality=Column vector (2-D)
  Reshape2 : Reshape  OutputDimensionality=Customize  OutputDimensions=[3,6]
  Reshape3 : Reshape  OutputDimensionality=Customize  OutputDimensions=[3,4]
  Selector{,1..3} (4 alike) : Selector  NumberOfDimensions=2  InputPortWidth=3  IndexOptions=Index vector (dialog),Index vector (dialog)  Indices=[1 3],1  OutputSizes=1,1
  Selector10 : Selector  NumberOfDimensions=2  InputPortWidth=3  IndexOptions=Index vector (dialog),Index vector (dialog)  Indices=[1 3],6  OutputSizes=1,1
  Selector11 : Selector  NumberOfDimensions=2  InputPortWidth=3  IndexOptions=Index vector (dialog),Index vector (dialog)  Indices=[1 3],6  OutputSizes=1,1
  Selector4 : Selector  NumberOfDimensions=2  InputPortWidth=3  IndexOptions=Index vector (dialog),Index vector (dialog)  Indices=[1 3],3  OutputSizes=1,1
  Selector5 : Selector  NumberOfDimensions=2  InputPortWidth=3  IndexOptions=Index vector (dialog),Index vector (dialog)  Indices=[1 3],3  OutputSizes=1,1
  Selector6 : Selector  NumberOfDimensions=2  InputPortWidth=3  IndexOptions=Index vector (dialog),Index vector (dialog)  Indices=[1 3],4  OutputSizes=1,1
  Selector7 : Selector  NumberOfDimensions=2  InputPortWidth=3  IndexOptions=Index vector (dialog),Index vector (dialog)  Indices=[1 3],4  OutputSizes=1,1
  Selector8 : Selector  NumberOfDimensions=2  InputPortWidth=3  IndexOptions=Index vector (dialog),Index vector (dialog)  Indices=[1 3],5  OutputSizes=1,1
  Selector9 : Selector  NumberOfDimensions=2  InputPortWidth=3  IndexOptions=Index vector (dialog),Index vector (dialog)  Indices=[1 3],5  OutputSizes=1,1
  Sum : Sum  Inputs=+-
  Sum{1..2,4..5} (4 alike) : Sum
  Sum3 : Sum  Inputs=+-
  F_MB : Outport
  F_SP : Outport  Port=2
  wires:
  Gain/1 -> Product/1
  Dot Product/1 -> ?
  Demux/6 -> Mux1/6
  Demux1/1 -> Mux5/1
  A_SP/1 -> Product4/2
  Mux5/1 -> Reshape4/1
  N_MB/1 -> Selector1/1, Selector3/1, Selector5/1, Selector7/1, Selector11/1, Product3/1, Selector9/1
  Dot Product1/1 -> Product6/1, Product4/3
  [S_B] -> Mux3/6
  Selector1/1 -> Dot Product/2
  [S_B] -> Mux3/2
  [SB_MB] -> Selector/1, Selector2/1, Selector4/1, Selector6/1, Selector8/1, Product1/1, Selector10/1
  Selector6/1 -> Dot Product4/1
  Gain5/1 -> Product6/2
  [SB_SP] -> Product5/1, Dot Product1/1
  Selector9/1 -> Dot Product5/2
  Selector8/1 -> Dot Product5/1
  Sum1/1 -> Product3/2
  Selector7/1 -> Dot Product4/2
  [S_B] -> Mux4/4
  Constant1/1 -> Sum3/1
  Demux1/5 -> Mux5/5
  Selector10/1 -> Dot Product6/1
  Demux1/4 -> Mux5/4
  Demux1/10 -> Mux6/4
  Gain1/1 -> Product2/2
  Selector11/1 -> Dot Product6/2
  Demux/8 -> Mux2/2
  Selector2/1 -> Dot Product2/1
  Demux/3 -> Mux1/3
  Demux1/6 -> Mux5/6
  Demux1/7 -> Mux6/1
  Reshape5/1 -> [RD_SP]
  Demux/5 -> Mux1/5
  Demux/7 -> Mux2/1
  [S_B] -> Mux4/1
  Product4/1 -> F_SP/1
  R_D/1 -> Demux1/1
  Demux/9 -> Mux2/3
  Selector/1 -> Dot Product/1
  [S_B] -> Mux3/1
  Demux/10 -> Mux2/4
  [S_B] -> Mux4/2
  SB/1 -> [S_B]
  [S_B] -> Mux3/4
  Reshape3/1 -> [SB_SP]
  Mux4/1 -> Reshape3/1
  [S_B] -> Mux3/3
  Selector4/1 -> Dot Product3/1
  Sum2/1 -> Product/4
  Product5/1 -> Sum5/1
  Demux1/9 -> Mux6/3
  Mux3/1 -> Reshape2/1
  Gain6/1 -> Sum4/2
  P/1 -> Demux/1
  Mux2/1 -> Reshape1/1
  Mux1/1 -> Reshape/1
  [S_B] -> Mux4/3
  Gain4/1 -> Product4/1
  Demux/4 -> Mux1/4
  n_SP/1 -> Dot Product1/2, Product7/1
  Selector5/1 -> Dot Product3/2
  [P_MB] -> Gain/1
  Product3/1 -> Sum2/2
  Reshape4/1 -> [RD_MB]
  Sum3/1 -> Product5/2
  Product6/1 -> Sum4/1
  Sum5/1 -> Product4/4
  Demux1/2 -> Mux5/2
  Demux1/3 -> Mux5/3
  Demux1/8 -> Mux6/2
  Sum4/1 -> Product7/2
  Rs_SP/1 -> Gain5/1, Sum3/2
  Product7/1 -> Sum5/2
  Selector3/1 -> Dot Product2/2
  Product2/1 -> Sum1/1
  [RD_MB] -> Gain2/1
  Gain2/1 -> Sum1/2
  Constant/1 -> Sum/1
  Reshape2/1 -> [SB_MB]
  RS_MB/1 -> Gain1/1, Sum/2
  Reshape1/1 -> [P_SP]
  Reshape/1 -> [P_MB]
  Product1/1 -> Sum2/1
  A_MB/1 -> Product/2
  [S_B] -> Mux3/5
  Mux6/1 -> Reshape5/1
  Sum/1 -> Product1/2
  Demux/1 -> Mux1/1
  Demux/2 -> Mux1/2
  Product/1 -> F_MB/1
  [P_SP] -> Gain4/1
  [RD_SP] -> Gain6/1

== system Quaternions_Method/Enviroment1/Solar Radiation Perturbation/Sum forces ==
  Input : Inport
  r_SP1 : Inport  Port=2
  r_SP2 : Inport  Port=3
  Cross Product : matrix_library/Cross Product
      settings: SourceProductBaseCode=SL
  Cross Product1 : matrix_library/Cross Product
      settings: SourceProductBaseCode=SL
  Cross Product2 : matrix_library/Cross Product
      settings: SourceProductBaseCode=SL
  Sum : Sum  Inputs=+++
  Out1 : Outport
  wires:
  Input/1 -> Cross Product/2, Cross Product1/2, Cross Product2/2
  ? -> Cross Product2/1
  r_SP2/1 -> Cross Product1/1
  Cross Product2/1 -> Sum/3
  Cross Product/1 -> Sum/1
  Cross Product1/1 -> Sum/2
  r_SP1/1 -> Cross Product/1

== system Quaternions_Method/Enviroment1/Solar Radiation Perturbation/Sun position body ==
  A_B_N : Inport
  Clock : Clock
  Constant : Constant  Value=2*pi
  Constant1 : Constant  Value=365*24*60*60
  Constant2 : Constant  Value=23.45
  Degrees to Radians : simulink_extras/Transformations/Degrees to Radians
  MatrixMultiply : Product  Multiplication=Matrix(*)
  Mux : Mux  Inputs=3
  Product{,1..3} (4 alike) : Product
  Reciprocal : Product  Inputs=1
  Sin : Trigonometry  Operator=cos
  Sin1 : Trigonometry
  Sin2 : Trigonometry  Operator=cos
  Sin3 : Trigonometry
  S_B : Outport
  wires:
  Product3/1 -> Mux/3
  Degrees to Radians/1 -> Sin3/1, Sin2/1
  Constant1/1 -> Reciprocal/1
  Sin2/1 -> Product2/2
  Product/1 -> Product1/1  "n"
  Constant2/1 -> Degrees to Radians/1
  Product1/1 -> Sin/1, Sin1/1  "n*t"
  Product2/1 -> Mux/2
  Sin3/1 -> Product3/2
  Clock/1 -> Product1/2
  Sin1/1 -> Product3/1, Product2/1
  Constant/1 -> Product/1
  Sin/1 -> Mux/1
  Reciprocal/1 -> Product/2
  Mux/1 -> MatrixMultiply/2
  A_B_N/1 -> MatrixMultiply/1
  MatrixMultiply/1 -> S_B/1

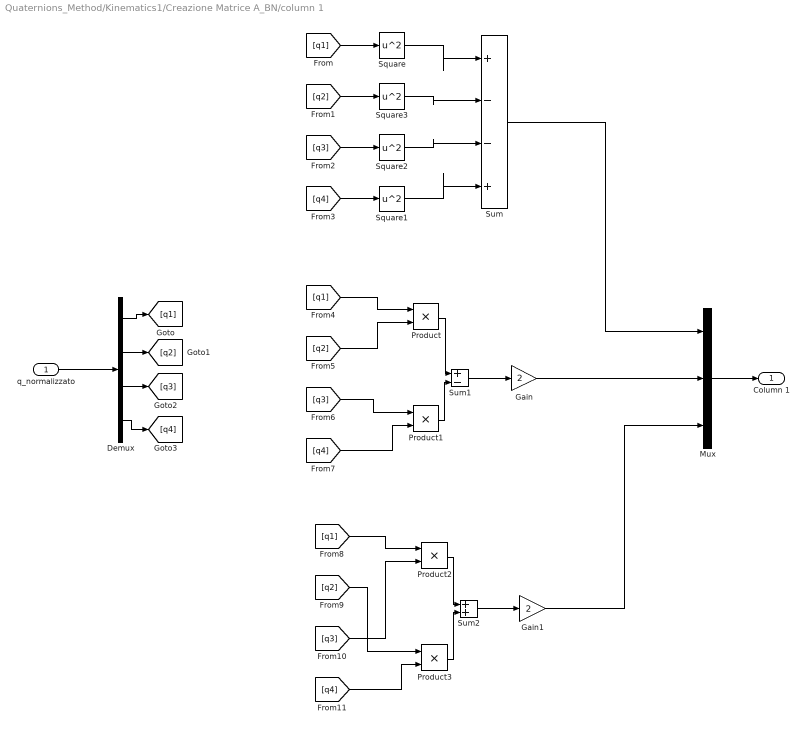
== system Quaternions_Method/Kinematics1/Creazione Matrice A_BN/column 1 ==
  q_normalizzato : Inport
  Demux : Demux
  Gain : Gain  Gain=2
  Gain1 : Gain  Gain=2
  Mux : Mux  Inputs=3
  Product{,1..3} (4 alike) : Product
  Square{,1..3} (4 alike) : Math  Operator=square  SaturateOnIntegerOverflow=on
  Sum : Sum  Inputs=|+|-|-|+|
  Sum1 : Sum  Inputs=|+|-|
  Sum2 : Sum  Inputs=|+|+|
  Column 1 : Outport
  wires:
  Demux/4 -> [q4]
  Demux/1 -> [q1]
  q_normalizzato/1 -> Demux/1
  Demux/3 -> [q3]
  Demux/2 -> [q2]
  [q1] -> Square/1
  [q2] -> Square3/1
  [q3] -> Square2/1
  [q4] -> Square1/1
  Square3/1 -> Sum/2
  Square/1 -> Sum/1
  Square1/1 -> Sum/4
  Square2/1 -> Sum/3
  [q4] -> Product1/2
  [q1] -> Product/1
  [q2] -> Product/2
  [q3] -> Product1/1
  Product/1 -> Sum1/1
  Product1/1 -> Sum1/2
  Sum1/1 -> Gain/1
  [q4] -> Product3/2
  [q1] -> Product2/1
  Product3/1 -> Sum2/2
  Product2/1 -> Sum2/1
  Sum2/1 -> Gain1/1
  [q3] -> Product2/2
  [q2] -> Product3/1
  Sum/1 -> Mux/1
  Gain/1 -> Mux/2
  Gain1/1 -> Mux/3
  Mux/1 -> Column 1/1

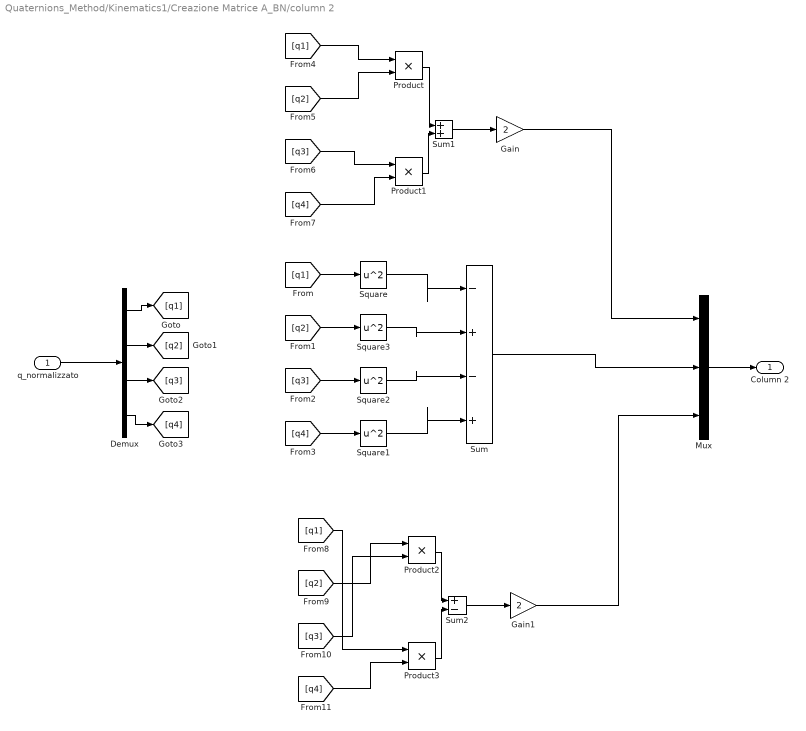
== system Quaternions_Method/Kinematics1/Creazione Matrice A_BN/column 2 ==
  q_normalizzato : Inport
  Demux : Demux
  Gain : Gain  Gain=2
  Gain1 : Gain  Gain=2
  Mux : Mux  Inputs=3
  Product{,1..3} (4 alike) : Product
  Square{,1..3} (4 alike) : Math  Operator=square  SaturateOnIntegerOverflow=on
  Sum : Sum  Inputs=|-|+|-|+|
  Sum1 : Sum  Inputs=|+|+|
  Sum2 : Sum  Inputs=|+|-|
  Column 2 : Outport
  wires:
  Demux/4 -> [q4]
  Demux/1 -> [q1]
  q_normalizzato/1 -> Demux/1
  Demux/3 -> [q3]
  Demux/2 -> [q2]
  Mux/1 -> Column 2/1
  Gain1/1 -> Mux/3
  Product2/1 -> Sum2/1
  Product3/1 -> Sum2/2
  Sum2/1 -> Gain1/1
  Sum1/1 -> Gain/1
  [q2] -> Product/2
  [q3] -> Product1/1
  [q4] -> Product1/2
  Product/1 -> Sum1/1
  Gain/1 -> Mux/1
  [q1] -> Product/1
  Product1/1 -> Sum1/2
  Sum/1 -> Mux/2
  [q1] -> Square/1
  Square1/1 -> Sum/4
  Square3/1 -> Sum/2
  [q4] -> Square1/1
  Square2/1 -> Sum/3
  [q2] -> Square3/1
  [q3] -> Square2/1
  Square/1 -> Sum/1
  [q2] -> Product2/1
  [q3] -> Product2/2
  [q1] -> Product3/1
  [q4] -> Product3/2

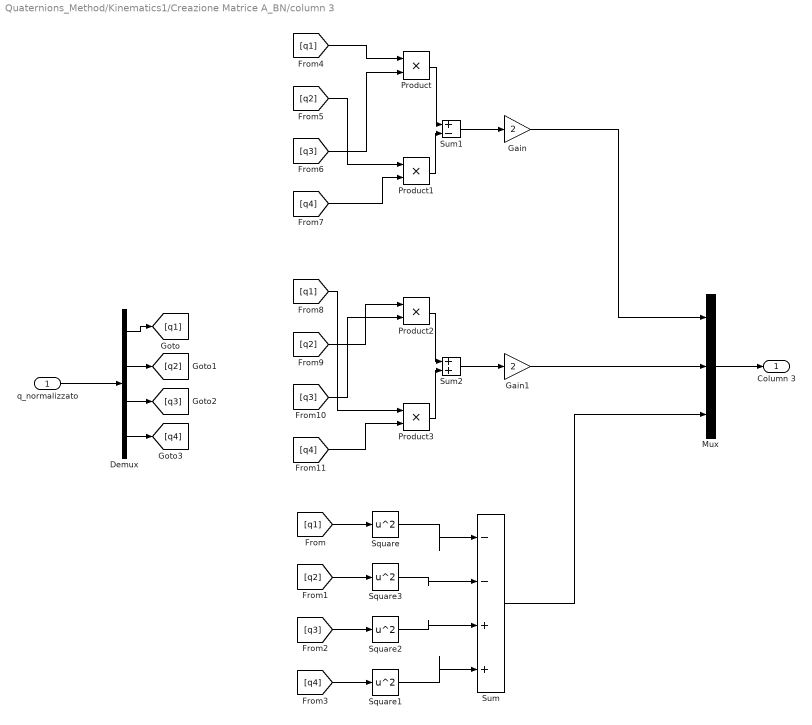
== system Quaternions_Method/Kinematics1/Creazione Matrice A_BN/column 3 ==
  q_normalizzato : Inport
  Demux : Demux
  Gain : Gain  Gain=2
  Gain1 : Gain  Gain=2
  Mux : Mux  Inputs=3
  Product{,1..3} (4 alike) : Product
  Square{,1..3} (4 alike) : Math  Operator=square  SaturateOnIntegerOverflow=on
  Sum : Sum  Inputs=|-|-|+|+|
  Sum1 : Sum  Inputs=|+|-|
  Sum2 : Sum  Inputs=|+|+|
  Column 3 : Outport
  wires:
  Demux/4 -> [q4]
  Demux/1 -> [q1]
  q_normalizzato/1 -> Demux/1
  Demux/3 -> [q3]
  Demux/2 -> [q2]
  Gain/1 -> Mux/1
  Product1/1 -> Sum1/2
  [q4] -> Product1/2
  Product/1 -> Sum1/1
  Mux/1 -> Column 3/1
  [q1] -> Product/1
  Sum1/1 -> Gain/1
  [q1] -> Square/1
  Square2/1 -> Sum/3
  Square3/1 -> Sum/2
  [q4] -> Square1/1
  Square1/1 -> Sum/4
  Square/1 -> Sum/1
  Sum/1 -> Mux/3
  [q3] -> Square2/1
  [q2] -> Square3/1
  [q2] -> Product2/1
  Product3/1 -> Sum2/2
  Gain1/1 -> Mux/2
  Sum2/1 -> Gain1/1
  Product2/1 -> Sum2/1
  [q3] -> Product2/2
  [q4] -> Product3/2
  [q1] -> Product3/1
  [q3] -> Product/2
  [q2] -> Product1/1

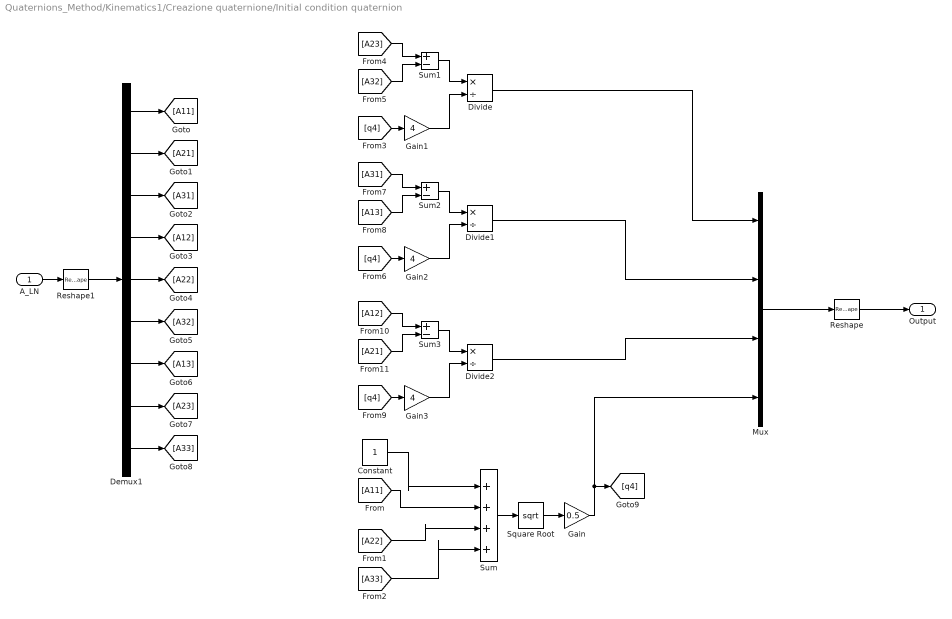
== system Quaternions_Method/Kinematics1/Creazione quaternione/Initial condition quaternion ==
  A_LN : Inport
  Constant : Constant
  Demux1 : Demux  Outputs=9
  Divide : Product  Inputs=*/
  Divide1 : Product  Inputs=*/
  Divide2 : Product  Inputs=*/
  Gain : Gain  Gain=0.5
  Gain1 : Gain  Gain=4
  Gain2 : Gain  Gain=4
  Gain3 : Gain  Gain=4
  Mux : Mux
  Reshape : Reshape  OutputDimensionality=Column vector (2-D)
  Reshape1 : Reshape  OutputDimensionality=Column vector (2-D)
  Square Root : Sqrt  SaturateOnIntegerOverflow=on
  Sum : Sum  Inputs=|+|+|+|+|
  Sum1 : Sum  Inputs=|+|-|
  Sum2 : Sum  Inputs=|+|-|
  Sum3 : Sum  Inputs=|+|-|
  Output : Outport
  wires:
  Demux1/3 -> [A31]
  Demux1/9 -> [A33]
  Demux1/1 -> [A11]
  A_LN/1 -> Reshape1/1
  Reshape1/1 -> Demux1/1
  Demux1/5 -> [A22]
  Demux1/2 -> [A21]
  Demux1/4 -> [A12]
  Demux1/6 -> [A32]
  Demux1/7 -> [A13]
  Demux1/8 -> [A23]
  Constant/1 -> Sum/1
  [A11] -> Sum/2
  [A22] -> Sum/3
  [A33] -> Sum/4
  Sum/1 -> Square Root/1
  Square Root/1 -> Gain/1
  Gain/1 -> Mux/4, [q4]
  [A23] -> Sum1/1
  [A32] -> Sum1/2
  Sum1/1 -> Divide/1
  [q4] -> Gain1/1
  Gain1/1 -> Divide/2
  Divide/1 -> Mux/1
  Divide1/1 -> Mux/2
  [A31] -> Sum2/1
  [A13] -> Sum2/2
  Sum2/1 -> Divide1/1
  [q4] -> Gain2/1
  Gain2/1 -> Divide1/2
  Divide2/1 -> Mux/3
  [A12] -> Sum3/1
  [A21] -> Sum3/2
  Sum3/1 -> Divide2/1
  [q4] -> Gain3/1
  Gain3/1 -> Divide2/2
  Mux/1 -> Reshape/1
  Reshape/1 -> Output/1

== system Quaternions_Method/Kinematics1/Creazione quaternione/Normalisation ==
  In1 : Inport
  Normalize Vector : vrlib/Utilities/Normalize Vector  maxzero=0
  Reshape : Reshape  OutputDimensionality=Column vector (2-D)
  Out1 : Outport
  wires:
  In1/1 -> Normalize Vector/1
  Normalize Vector/1 -> Reshape/1
  Reshape/1 -> Out1/1

== system Quaternions_Method/Kinematics1/Relative_Attitude/A_LN ==
  theta : Inport
  Constant : Constant  Value=ii
  M1 : Subsystem
  M2 : Subsystem
  MatrixMultiply : Product  Multiplication=Matrix(*)
  A_LN : Outport
  wires:
  theta/1 -> M1/1(Input)
  M1/1(Out1) -> MatrixMultiply/1
  M2/1(Out1) -> MatrixMultiply/2
  MatrixMultiply/1 -> A_LN/1
  Constant/1 -> M2/1(ii)

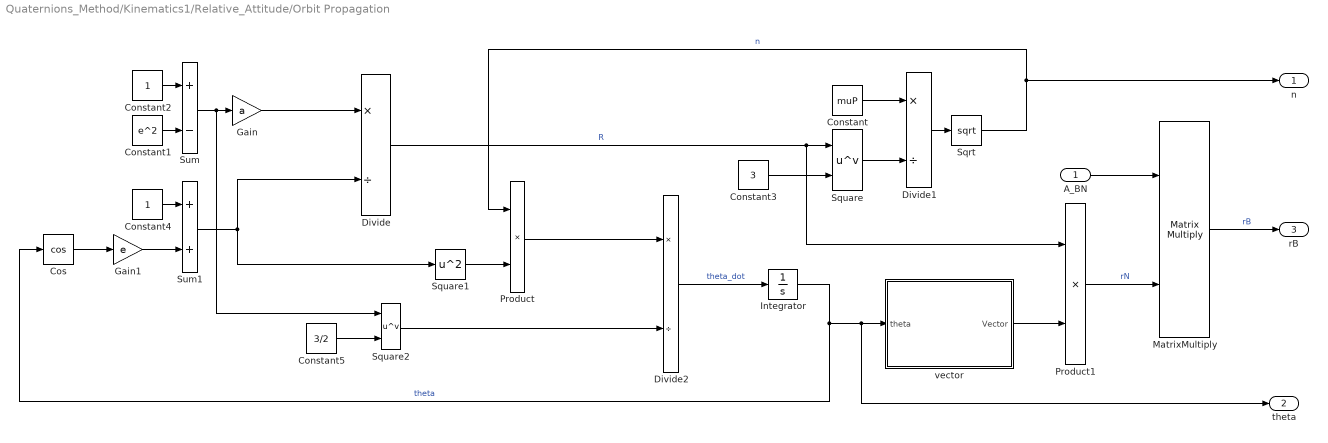
== system Quaternions_Method/Kinematics1/Relative_Attitude/Orbit Propagation ==
  A_BN : Inport
  Constant : Constant  Value=muP
  Constant1 : Constant  Value=e^2
  Constant2 : Constant
  Constant3 : Constant  Value=3
  Constant4 : Constant
  Constant5 : Constant  Value=3/2
  Cos : Trigonometry  Operator=cos
  Divide : Product  Inputs=*/
  Divide1 : Product  Inputs=*/
  Divide2 : Product  Inputs=*/
  Gain : Gain  Gain=a
  Gain1 : Gain  Gain=e
  Integrator : Integrator  InitialCondition=theta00
  MatrixMultiply : Product  Multiplication=Matrix(*)
  Product : Product
  Product1 : Product
  Sqrt : Sqrt  SaturateOnIntegerOverflow=on
  Square : Math  Operator=pow  SaturateOnIntegerOverflow=on
  Square1 : Math  Operator=square  SaturateOnIntegerOverflow=on
  Square2 : Math  Operator=pow  SaturateOnIntegerOverflow=on
  Sum : Sum  Inputs=+-
  Sum1 : Sum
  vector : Subsystem
  n : Outport
  theta : Outport  Port=2
  rB : Outport  Port=3
  wires:
  Constant2/1 -> Sum/1
  Constant1/1 -> Sum/2
  Sum/1 -> Square2/1, Gain/1
  Gain/1 -> Divide/1
  Constant4/1 -> Sum1/1
  Sum1/1 -> Square1/1, Divide/2
  Gain1/1 -> Sum1/2
  Cos/1 -> Gain1/1
  Integrator/1 -> Cos/1, theta/1, vector/1(theta)  "theta"
  Divide1/1 -> Sqrt/1
  Constant/1 -> Divide1/1
  Square/1 -> Divide1/2
  Divide/1 -> Product1/1, Square/1  "R"
  Constant3/1 -> Square/2
  Sqrt/1 -> Product/1, n/1  "n"
  Square1/1 -> Product/2
  Constant5/1 -> Square2/2
  Product/1 -> Divide2/1
  Divide2/1 -> Integrator/1  "theta_dot"
  vector/1(Vector) -> Product1/2
  A_BN/1 -> MatrixMultiply/1
  Product1/1 -> MatrixMultiply/2  "rN"
  MatrixMultiply/1 -> rB/1  "rB"
  Square2/1 -> Divide2/2

== system Quaternions_Method/Kinematics1/Relative_Attitude/A_LN/M1 ==
  Input : Inport
  Constant{1..2,4..5} (4 alike) : Constant  Value=0
  Constant3 : Constant
  Cos : Trigonometry  Operator=cos
  Cos1 : Trigonometry
  Cos2 : Trigonometry  Operator=cos
  Cos3 : Trigonometry
  Matrix Concatenate : Concatenate  NumInputs=3  Mode=Multidimensional array  ConcatenateDimension=2
  Multiply : Gain  Gain=-1
  Mux : Mux  Inputs=3
  Mux1 : Mux  Inputs=3
  Mux2 : Mux  Inputs=3
  Reshape : Reshape  OutputDimensionality=Column vector (2-D)
  Reshape1 : Reshape  OutputDimensionality=Column vector (2-D)
  Reshape2 : Reshape  OutputDimensionality=Column vector (2-D)
  Out1 : Outport
  wires:
  Multiply/1 -> Mux/2
  Cos/1 -> Mux/1
  Constant1/1 -> Mux/3
  Constant2/1 -> Mux1/3
  Input/1 -> Cos/1, Cos1/1, Cos3/1, Cos2/1
  Matrix Concatenate/1 -> Out1/1
  Cos3/1 -> Mux1/1
  Constant5/1 -> Mux2/1
  Cos2/1 -> Mux1/2
  Constant3/1 -> Mux2/3
  Constant4/1 -> Mux2/2
  Cos1/1 -> Multiply/1
  Mux/1 -> Reshape/1
  Reshape/1 -> Matrix Concatenate/1
  Reshape1/1 -> Matrix Concatenate/2
  Mux1/1 -> Reshape1/1
  Mux2/1 -> Reshape2/1
  Reshape2/1 -> Matrix Concatenate/3

== system Quaternions_Method/Kinematics1/Relative_Attitude/A_LN/M2 ==
  ii : Inport
  Constant{1..4} (4 alike) : Constant  Value=0
  Constant5 : Constant
  Cos : Trigonometry  Operator=cos
  Cos1 : Trigonometry
  Cos2 : Trigonometry  Operator=cos
  Cos3 : Trigonometry
  Matrix Concatenate : Concatenate  NumInputs=3  Mode=Multidimensional array  ConcatenateDimension=2
  Multiply : Gain  Gain=-1
  Mux : Mux  Inputs=3
  Mux1 : Mux  Inputs=3
  Mux2 : Mux  Inputs=3
  Reshape : Reshape  OutputDimensionality=Column vector (2-D)
  Reshape1 : Reshape  OutputDimensionality=Column vector (2-D)
  Reshape2 : Reshape  OutputDimensionality=Column vector (2-D)
  Out1 : Outport
  wires:
  Matrix Concatenate/1 -> Out1/1
  Constant5/1 -> Mux2/1
  Constant3/1 -> Mux2/3
  Constant4/1 -> Mux2/2
  Cos1/1 -> Multiply/1
  Constant1/1 -> Mux/1
  Cos/1 -> Mux/2
  Multiply/1 -> Mux/3
  Constant2/1 -> Mux1/1
  Cos3/1 -> Mux1/2
  Cos2/1 -> Mux1/3
  ii/1 -> Cos2/1, Cos/1, Cos1/1, Cos3/1
  Mux2/1 -> Reshape/1
  Reshape/1 -> Matrix Concatenate/1
  Mux/1 -> Reshape1/1
  Reshape1/1 -> Matrix Concatenate/2
  Reshape2/1 -> Matrix Concatenate/3
  Mux1/1 -> Reshape2/1

== system Quaternions_Method/Kinematics1/Relative_Attitude/Orbit Propagation/vector ==
  theta : Inport
  Constant : Constant  Value=ii
  Cos : Trigonometry  Operator=cos
  Cos1 : Trigonometry
  Cos2 : Trigonometry  Operator=cos
  Cos3 : Trigonometry
  Cos4 : Trigonometry
  Mux : Mux  Inputs=3
  Product : Product
  Product1 : Product
  Vector : Outport
  wires:
  Mux/1 -> Vector/1
  Cos/1 -> Mux/1
  Cos1/1 -> Product/1
  Cos2/1 -> Product/2
  Product/1 -> Mux/2
  Cos4/1 -> Product1/2
  Product1/1 -> Mux/3
  Cos3/1 -> Product1/1
  theta/1 -> Cos3/1, Cos1/1, Cos/1
  Constant/1 -> Cos4/1, Cos2/1

== matlab function Quaternions_Method/Kinematics1/Creazione quaternione/Creation matrix [OM] ==
  data: om_x input; OM output; om_y input; om_z input
function OM  = fcn(om_x, om_y, om_z)

OM = [0 om_z -om_y om_x; 
      -om_z 0 om_x om_y; 
      om_y -om_x 0 om_z;
      -om_x -om_y -om_z 0];

end
